simulink model "ZadanieCsim"  (R2023b)
settings: Solver=VariableStepAuto  StartTime=0.0  StopTime=10.0  RelTol=1e-3
settings Model: Creator=Filip  LastModifiedBy=Henka

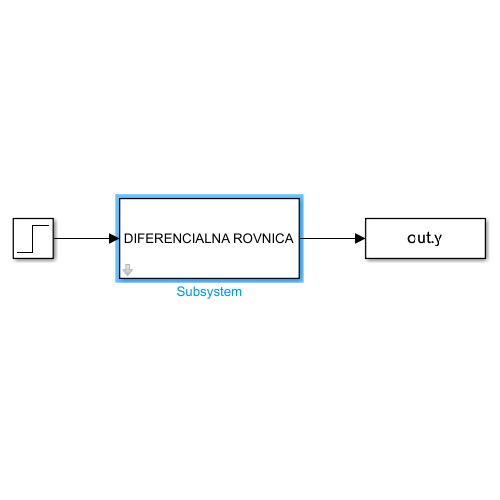
[thumbnail: Simulink's stored preview of the top-level diagram]
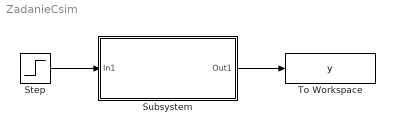
== system ZadanieCsim ==
  Step : Step  Time=0  SampleTime=0
  Subsystem : Subsystem  mask{a0=3, a1=2, y0=0.05, yd0=0}
      mask Display: disp('DIFERENCIALNA ROVNICA');
  To Workspace : ToWorkspace  VariableName=y  SaveFormat=Timeseries  SampleTime=-1
  wires:
  Step/1 -> Subsystem/1(In1)
  Subsystem/1(Out1) -> To Workspace/1

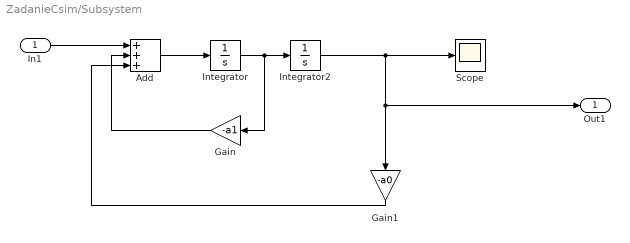
== system ZadanieCsim/Subsystem ==
  In1 : Inport
  Add : Sum  Inputs=+++
  Gain : Gain  Gain=-a1
  Gain1 : Gain  Gain=-a0
  Integrator : Integrator  InitialCondition=yd0
  Integrator2 : Integrator  InitialCondition=y0
  Scope : Scope
  Out1 : Outport
  wires:
  Integrator/1 -> Gain/1, Integrator2/1
  Integrator2/1 -> Scope/1, Out1/1, Gain1/1
  In1/1 -> Add/1
  Gain1/1 -> Add/3
  Add/1 -> Integrator/1
  Gain/1 -> Add/2
